simulink model "sixth_harmonic_makale"  (R2013a)
settings: Solver=ode4  StartTime=0.0  StopTime=0.5  FixedStep=Ts  RelTol=1e-3
values from neighbouring files (symbols this model uses):
  Lload = Xload/wout_fund    [acemp_sixth.m]    (also in immd_base_varyingmod.m = Xload/wout; immd_design_elen.m = Xload/wout; immd_efficiency.m = Xload/wout; immd_simulation_base.m = Xload/wout)
  ma1 = 0.8    [acemp_sixth.m]
  ma3 = 0.3    [acemp_sixth.m]
  Rload = Zload*pf    [acemp_sixth.m]    (also in immd_base_varyingmod.m; immd_design_elen.m; immd_efficiency.m; immd_simulation_base.m)
  Ts = 1e-6    (= 1e-06)    [acemp_sixth.m]    (also in immd_base_varyingmod.m = 1e-05; immd_design_elen.m; immd_efficiency.m; immd_simulation_base.m)
  wout_fund = 2*pi*fout_fund    (= 314.159265359)    [acemp_sixth.m]
  wout_three = 2*pi*fout_three    (= 942.477796077)    [acemp_sixth.m]
undefined symbols (not defined in the file or in its folder): phase3, phasegrid
libraries: powerlib x84, powerlib_meascontrol x61, simulink x2
settings Model: Creator=ugurm  LastModifiedBy=ugurm

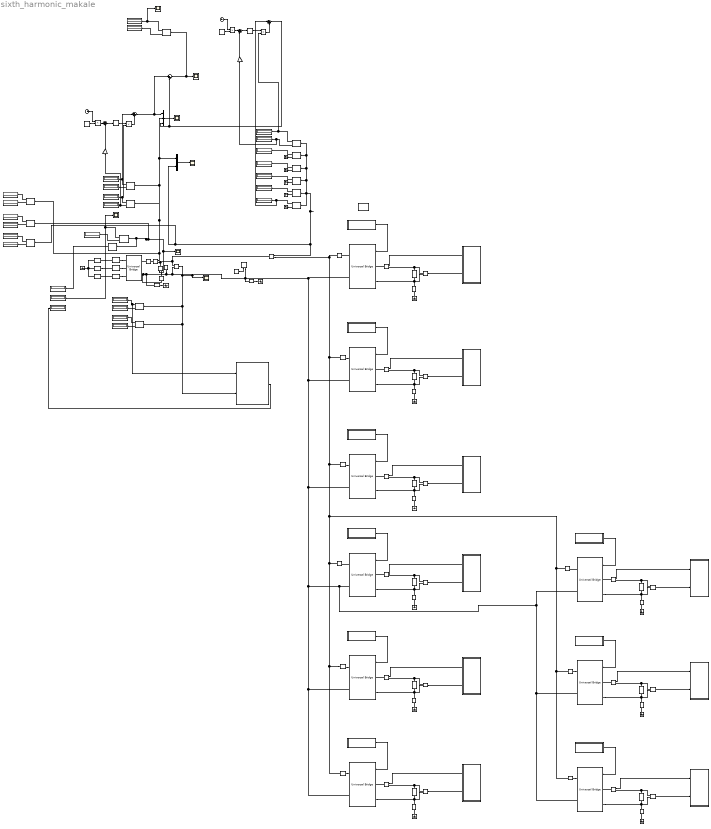
== system sixth_harmonic_makale ==
  AC Voltage Source : powerlib/Electrical Sources/AC Voltage Source  Amplitude=230*sqrt(2)  Phase=phasegrid  Frequency=50  SampleTime=Ts  Measurements=None
  AC Voltage Source1 : powerlib/Electrical Sources/AC Voltage Source  Amplitude=230*sqrt(2)  Phase=-120+phasegrid  Frequency=50  SampleTime=Ts  Measurements=None
  AC Voltage Source2 : powerlib/Electrical Sources/AC Voltage Source  Amplitude=230*sqrt(2)  Phase=120+phasegrid  Frequency=50  SampleTime=Ts  Measurements=None
  Clock : Clock
  Clock1 : Clock
  Constant : Constant  Value=2*pi*300
  Constant1 : Constant  Value=538
  Constant2 : Constant  Value=2*pi*300
  Display{1..20,23,26..28} (24 alike) : Display
  Fourier1 : powerlib_meascontrol/Measurements/Fourier  Freq=50  n=0  InInit=[0, 0]  Ts=Ts
  Fourier10 : powerlib_meascontrol/Measurements/Fourier  Freq=fout_fund  n=6  InInit=[0, 0]  Ts=Ts
  Fourier11 : powerlib_meascontrol/Measurements/Fourier  Freq=50  n=2  InInit=[0, 0]  Ts=Ts
  Fourier12 : powerlib_meascontrol/Measurements/Fourier  Freq=50  n=2  InInit=[0, 0]  Ts=Ts
  Fourier13 : powerlib_meascontrol/Measurements/Fourier  Freq=50  n=0  InInit=[0, 0]  Ts=Ts
  Fourier14 : powerlib_meascontrol/Measurements/Fourier  Freq=50  n=2  InInit=[0, 0]  Ts=Ts
  Fourier15 : powerlib_meascontrol/Measurements/Fourier  Freq=50  n=6  InInit=[0, 0]  Ts=Ts
  Fourier2 : powerlib_meascontrol/Measurements/Fourier  Freq=50  n=6  InInit=[0, 0]  Ts=Ts
  Fourier3 : powerlib_meascontrol/Measurements/Fourier  Freq=fout_fund  n=6  InInit=[0, 0]  Ts=Ts
  Fourier4 : powerlib_meascontrol/Measurements/Fourier  Freq=fout_fund  n=1  InInit=[0, 0]  Ts=Ts
  Fourier5 : powerlib_meascontrol/Measurements/Fourier  Freq=fout_fund  n=0  InInit=[0, 0]  Ts=Ts
  Fourier6 : powerlib_meascontrol/Measurements/Fourier  Freq=fout_fund  n=3  InInit=[0, 0]  Ts=Ts
  Fourier7 : powerlib_meascontrol/Measurements/Fourier  Freq=fout_fund  n=2  InInit=[0, 0]  Ts=Ts
  Fourier8 : powerlib_meascontrol/Measurements/Fourier  Freq=fout_fund  n=6  InInit=[0, 0]  Ts=Ts
  Fourier9 : powerlib_meascontrol/Measurements/Fourier  Freq=fout_fund  n=4  InInit=[0, 0]  Ts=Ts
  Gain : Gain  Gain=pi/180
  Gain1 : Gain  Gain=pi/180
  Gate drive 1 : Subsystem
  Gate drive 2 : Subsystem
  Gate drive 3 : Subsystem
  Gate drive 4 : Subsystem
  Gate drive 5 : Subsystem
  Gate drive 6 : Subsystem
  Gate drive 7 : Subsystem
  Gate drive 8 : Subsystem
  Gate drive 9 : Subsystem
  Ground{1..12} (12 alike) : powerlib/Elements/Ground  LConnTagsString=a
  Idc_m{1..21} (21 alike) : powerlib/Measurements/Current Measurement  PhasorSimulation=off  OutputType=Complex  PSBequivalent=0
  Mux1 : Mux  Inputs=3
  Mux2 : Mux  Inputs=2
  Product{,1..3} (4 alike) : Product
  RMS : powerlib_meascontrol/Measurements/RMS  TrueRMS=on  Freq=50  RMSInit=0  Ts=0
  Scope{1..7} (7 alike) : Scope
      Scope1 settings: YMin=-25  YMax=50  SaveName=idc1
      Scope2 settings: YMin=52.5  YMax=100  SaveName=idc
      Scope3 settings: YMin=0  YMax=100  SaveName=idc2
      Scope4 settings: YMin=440  YMax=650  SaveName=makalee
      Scope5 settings: YMin=0  YMax=25  SaveName=idc4
      Scope6 settings: YMin=0  YMax=25  SaveName=idc5
      Scope7 settings: YMin=440  YMax=650  SaveName=makalee1
  Series RLC Branch{1..2,5,7..8,12..14,17,24..25} (11 alike) : powerlib/Elements/Series RLC Branch  LConnTagsString=__new0  RConnTagsString=__new0  BranchType=R  Resistance=1e12  Inductance=Lload  SetiL0=off  InitialCurrent=0  Capacitance=1e-6  Setx0=off  InitialVoltage=0  Measurements=None
  Series RLC Branch{3..4,6,9..11,22..23,26} (9 alike) : powerlib/Elements/Series RLC Branch  LConnTagsString=__new0  RConnTagsString=__new0  BranchType=RL  Resistance=Rload  Inductance=Lload  SetiL0=off  InitialCurrent=0  Capacitance=1e-6  Setx0=off  InitialVoltage=0  Measurements=None
  Series RLC Branch15 : powerlib/Elements/Series RLC Branch  LConnTagsString=__new0  RConnTagsString=__new0  BranchType=R  Resistance=22.97  Inductance=Lload  SetiL0=off  InitialCurrent=0  Capacitance=1e-6  Setx0=off  InitialVoltage=0  Measurements=None
  Series RLC Branch16 : powerlib/Elements/Series RLC Branch  LConnTagsString=__new0  RConnTagsString=__new0  BranchType=RC  Resistance=1e-9  Inductance=Lload  SetiL0=off  InitialCurrent=0  Capacitance=2e-3  Setx0=off  InitialVoltage=0  Measurements=None
  Series RLC Branch18 : powerlib/Elements/Series RLC Branch  LConnTagsString=__new0  RConnTagsString=__new0  BranchType=RL  Resistance=1e-6  Inductance=1e-9  SetiL0=off  InitialCurrent=0  Capacitance=100e-6  Setx0=off  InitialVoltage=0  Measurements=None
  Series RLC Branch19 : powerlib/Elements/Series RLC Branch  LConnTagsString=__new0  RConnTagsString=__new0  BranchType=RL  Resistance=1e-6  Inductance=1e-9  SetiL0=off  InitialCurrent=0  Capacitance=100e-6  Setx0=off  InitialVoltage=0  Measurements=None
  Series RLC Branch20 : powerlib/Elements/Series RLC Branch  LConnTagsString=__new0  RConnTagsString=__new0  BranchType=RL  Resistance=1e-6  Inductance=1e-9  SetiL0=off  InitialCurrent=0  Capacitance=100e-6  Setx0=off  InitialVoltage=0  Measurements=None
  Series RLC Branch21 : powerlib/Elements/Series RLC Branch  LConnTagsString=__new0  RConnTagsString=__new0  BranchType=RL  Resistance=1e-6  Inductance=1e-3  SetiL0=off  InitialCurrent=0  Capacitance=100e-6  Setx0=off  InitialVoltage=0  Measurements=None
  Subsystem : Subsystem
  Subsystem1 : Subsystem
  Subsystem2 : Subsystem
  Subsystem3 : Subsystem
  Subsystem4 : Subsystem
  Subsystem5 : Subsystem
  Subsystem6 : Subsystem
  Subsystem7 : Subsystem
  Subsystem8 : Subsystem
  Subsystem9 : Subsystem
  Sum{,1..3} (4 alike) : Sum  Inputs=|++
  Sum4 : Sum  Inputs=|+-
  Terminator{4..7,9} (5 alike) : Terminator
  Trigonometric Function : Trigonometry
  Trigonometric Function1 : Trigonometry
  Universal Bridge{1,3..10} (9 alike) : powerlib/Power Electronics/Universal Bridge  Arms=2  SnubberResistance=1e5  SnubberCapacitance=inf  Device=IGBT / Diodes  Ron=1e-6  Lon=0  ForwardVoltages="[  0  0  ]"  ForwardVoltage=0  GTOparameters=[ 10e-6 , 20e-6 ]  IGBTparameters=[0,0]  Measurements=None  Measurements_2=None  converterType=Rectifier
  Universal Bridge2 : powerlib/Power Electronics/Universal Bridge  Arms=3  SnubberResistance=1e5  SnubberCapacitance=inf  Device=Diodes  Ron=1e-6  Lon=0  ForwardVoltages="[  0  0  ]"  ForwardVoltage=0  GTOparameters=[ 10e-6 , 20e-6 ]  IGBTparameters=[0,0]  Measurements=None  Measurements_2=None  converterType=Rectifier
  Vdc2 : powerlib/Electrical Sources/Controlled Voltage Source  Initialize=off  Source_Type=DC  Amplitude=200  Phase=0  Frequency=0  Measurements=None
  Vdc_m{1..10} (10 alike) : powerlib/Measurements/Voltage Measurement  PhasorSimulation=off  OutputType=Complex  PSBequivalent=0
  cap_6 : Display
  cap_rms : Display
  perc_rip : Display
  powergui : powerlib/powergui  Priority=1  SimulationMode=Discrete  SolverType=Tustin  SampleTime=Ts  frequency=60  SPID=off  DisableSnubberDevices=off  DisableRonSwitches=off  DisableVfSwitches=off  SwTol=0  Interpol=off  DisplayEquations=off  frequencyindice=0  Pbase=100e6  ErrMax=1e-4  Iterations=50  UnitsV=kV  UnitsW=MW  FunctionMessages=off  echomessages=off  HookPort=off  EnableUseOfTLC=off  x0status=blocks  RestoreLinks=warning  ResistiveCurrentMeasurement=off  Frange=[0:2:500]  Ylog=off  Xlog=on  ShowGrid=off  save=off  variable=ZData  structure=makalee1  ZoomFFT=off  StartTime=0.2  cycles=15  DisplayStyle=3  fundamental=50  FreqAxis=off  MaxFrequency=1000  frequencyindicesteady=1  RmsSteady=1  display=off  Ts=0  methode=off
  wires:
  Gate drive 1/1(gate1) -> Universal Bridge1/1
  Fourier4/1 -> Display1/1
  Fourier4/2 -> Terminator4/1
  Fourier5/2 -> Terminator5/1
  Fourier6/1 -> Display3/1
  Fourier6/2 -> Terminator6/1
  Fourier7/1 -> Display4/1
  Fourier7/2 -> Terminator7/1
  Idc_m7/1 -> Fourier8/1, Fourier9/1, Fourier6/1, Fourier7/1, Fourier5/1, Fourier4/1, Fourier14/1, Mux2/2
  Fourier9/1 -> Display6/1
  Fourier9/2 -> Terminator9/1
  Idc_m2/1 -> Subsystem/1(In1)
  Vdc_m2/1 -> Subsystem/2(In2)
  Gate drive 2/1(gate1) -> Universal Bridge3/1
  Idc_m3/1 -> Subsystem1/1(In1)
  Vdc_m5/1 -> Subsystem1/2(In2)
  Gate drive 4/1(gate1) -> Universal Bridge4/1
  Idc_m9/1 -> Subsystem2/1(In1)
  Vdc_m6/1 -> Subsystem2/2(In2)
  Constant1/1 -> Vdc2/1
  Vdc_m4/1 -> Scope4/1, Fourier13/1, Subsystem3/2(In2), Fourier15/1
  Fourier13/2 -> Display16/1
  Fourier15/1 -> Display28/1
  Fourier15/2 -> Display27/1
  Fourier1/1 -> Sum/1, Display8/1
  Fourier1/2 -> Display7/1
  Fourier2/1 -> Product/2, Display10/1
  Fourier2/2 -> Gain/1, Display9/1
  Mux2/1 -> Scope1/1
  Trigonometric Function/1 -> Product/1
  Product/1 -> Sum/2
  Clock/1 -> Product1/1
  Constant/1 -> Product1/2
  Product1/1 -> Sum1/1
  Gain/1 -> Sum1/2
  Sum1/1 -> Trigonometric Function/1
  Sum/1 -> Sum4/1, Mux1/1
  Mux1/1 -> Scope2/1
  Fourier5/1 -> Sum2/1, Display2/1
  Fourier8/1 -> Product2/2, Display5/1
  Fourier8/2 -> Gain1/1, Display23/1
  Trigonometric Function1/1 -> Product2/1
  Product2/1 -> Sum2/2
  Clock1/1 -> Product3/1
  Constant2/1 -> Product3/2
  Product3/1 -> Sum3/1
  Gain1/1 -> Sum3/2
  Sum3/1 -> Trigonometric Function1/1
  Sum2/1 -> Sum4/2, Mux1/3
  Sum4/1 -> Fourier3/1, Scope3/1
  Fourier3/1 -> Scope5/1, Display12/1
  Fourier3/2 -> Display11/1
  Idc_m5/1 -> Scope7/1, Fourier12/1, RMS/1, Fourier10/1
  Fourier10/1 -> Scope6/1, cap_6/1
  Fourier10/2 -> Display13/1
  RMS/1 -> cap_rms/1
  Fourier13/1 -> Subsystem3/1(In1), Display26/1
  Subsystem3/1(Out1) -> perc_rip/1
  Gate drive 3/1(gate1) -> Universal Bridge5/1
  Idc_m12/1 -> Subsystem4/1(In1)
  Vdc_m1/1 -> Subsystem4/2(In2)
  Gate drive 5/1(gate1) -> Universal Bridge6/1
  Idc_m13/1 -> Subsystem5/1(In1)
  Vdc_m3/1 -> Subsystem5/2(In2)
  Gate drive 6/1(gate1) -> Universal Bridge7/1
  Idc_m15/1 -> Subsystem6/1(In1)
  Vdc_m7/1 -> Subsystem6/2(In2)
  Gate drive 7/1(gate1) -> Universal Bridge8/1
  Idc_m17/1 -> Subsystem7/1(In1)
  Vdc_m8/1 -> Subsystem7/2(In2)
  Gate drive 8/1(gate1) -> Universal Bridge9/1
  Idc_m18/1 -> Subsystem8/1(In1)
  Vdc_m9/1 -> Subsystem8/2(In2)
  Gate drive 9/1(gate1) -> Universal Bridge10/1
  Idc_m20/1 -> Subsystem9/1(In1)
  Vdc_m10/1 -> Subsystem9/2(In2)
  Idc_m4/1 -> Fourier11/1, Fourier2/1, Mux1/2, Mux2/1, Fourier1/1
  Fourier11/2 -> Display14/1
  Fourier11/1 -> Display15/1
  Fourier12/2 -> Display17/1
  Fourier12/1 -> Display18/1
  Fourier14/2 -> Display19/1
  Fourier14/1 -> Display20/1
  connections:
  Universal Bridge1/RConn1 -- Idc_m1/RConn1
  Universal Bridge1/LConn2 -- Series RLC Branch2/LConn1 -- Vdc_m2/LConn2 -- Series RLC Branch6/RConn1
  Idc_m2/LConn1 -- Universal Bridge1/LConn1
  Series RLC Branch6/LConn1 -- Vdc_m2/LConn1 -- Idc_m2/RConn1
  Ground2/LConn1 -- Series RLC Branch2/RConn1
  Series RLC Branch10/RConn1 -- Series RLC Branch7/LConn1 -- Universal Bridge3/LConn2 -- Vdc_m5/LConn2
  Series RLC Branch10/LConn1 -- Vdc_m5/LConn1 -- Idc_m3/RConn1
  Ground1/LConn1 -- Series RLC Branch7/RConn1
  Idc_m3/LConn1 -- Universal Bridge3/LConn1
  Idc_m6/RConn1 -- Universal Bridge3/RConn1
  Series RLC Branch11/RConn1 -- Series RLC Branch12/LConn1 -- Universal Bridge4/LConn2 -- Vdc_m6/LConn2
  Series RLC Branch11/LConn1 -- Vdc_m6/LConn1 -- Idc_m9/RConn1
  Ground3/LConn1 -- Series RLC Branch12/RConn1
  Idc_m9/LConn1 -- Universal Bridge4/LConn1
  Idc_m11/RConn1 -- Universal Bridge4/RConn1
  Series RLC Branch1/RConn1 -- Ground4/LConn1
  Ground6/LConn1 -- AC Voltage Source2/LConn1 -- AC Voltage Source/LConn1 -- AC Voltage Source1/LConn1
  Series RLC Branch17/RConn1 -- Ground7/LConn1
  Series RLC Branch20/RConn1 -- AC Voltage Source2/RConn1
  AC Voltage Source1/RConn1 -- Series RLC Branch19/RConn1
  Series RLC Branch18/RConn1 -- AC Voltage Source/RConn1
  Series RLC Branch18/LConn1 -- Universal Bridge2/LConn1
  Series RLC Branch19/LConn1 -- Universal Bridge2/LConn2
  Series RLC Branch20/LConn1 -- Universal Bridge2/LConn3
  Vdc_m4/LConn1 -- Idc_m5/LConn1 -- Idc_m4/RConn1 -- Idc_m7/LConn1
  Series RLC Branch21/RConn1 -- Universal Bridge2/RConn1
  Idc_m4/LConn1 -- Series RLC Branch21/LConn1
  Idc_m5/RConn1 -- Series RLC Branch16/LConn1
  Series RLC Branch9/RConn1 -- Universal Bridge5/LConn2 -- Series RLC Branch8/LConn1 -- Vdc_m1/LConn2
  Idc_m12/RConn1 -- Series RLC Branch9/LConn1 -- Vdc_m1/LConn1
  Vdc_m3/LConn2 -- Series RLC Branch3/RConn1 -- Series RLC Branch13/LConn1 -- Universal Bridge6/LConn2
  Idc_m13/RConn1 -- Series RLC Branch3/LConn1 -- Vdc_m3/LConn1
  Vdc_m7/LConn2 -- Series RLC Branch4/RConn1 -- Series RLC Branch5/LConn1 -- Universal Bridge7/LConn2
  Idc_m15/RConn1 -- Series RLC Branch4/LConn1 -- Vdc_m7/LConn1
  Ground9/LConn1 -- Series RLC Branch5/RConn1
  Universal Bridge5/RConn1 -- Idc_m8/RConn1
  Ground5/LConn1 -- Series RLC Branch13/RConn1
  Ground8/LConn1 -- Series RLC Branch8/RConn1
  Idc_m12/LConn1 -- Universal Bridge5/LConn1
  Idc_m15/LConn1 -- Universal Bridge7/LConn1
  Idc_m13/LConn1 -- Universal Bridge6/LConn1
  Idc_m14/RConn1 -- Universal Bridge6/RConn1
  Idc_m10/RConn1 -- Universal Bridge7/RConn1
  Idc_m14/LConn1 -- Idc_m8/LConn1 -- Idc_m16/LConn1 -- Idc_m19/LConn1 -- Idc_m21/LConn1 -- Idc_m1/LConn1 -- Idc_m7/RConn1 -- Idc_m6/LConn1 -- Idc_m11/LConn1 -- Idc_m10/LConn1
  Universal Bridge7/RConn2 -- Universal Bridge8/RConn2 -- Universal Bridge9/RConn2 -- Universal Bridge10/RConn2 -- Universal Bridge5/RConn2 -- Universal Bridge3/RConn2 -- Series RLC Branch15/LConn1 -- Series RLC Branch16/RConn1 -- Universal Bridge2/RConn2 -- Series RLC Branch17/LConn1 -- Vdc_m4/LConn2 -- Series RLC Branch1/LConn1 -- Vdc2/LConn1 -- Universal Bridge1/RConn2 -- Universal Bridge4/RConn2 -- Universal Bridge6/RConn2
  Series RLC Branch26/RConn1 -- Universal Bridge8/LConn2 -- Series RLC Branch25/LConn1 -- Vdc_m8/LConn2
  Idc_m17/RConn1 -- Series RLC Branch26/LConn1 -- Vdc_m8/LConn1
  Vdc_m9/LConn2 -- Series RLC Branch22/RConn1 -- Series RLC Branch14/LConn1 -- Universal Bridge9/LConn2
  Idc_m18/RConn1 -- Series RLC Branch22/LConn1 -- Vdc_m9/LConn1
  Vdc_m10/LConn2 -- Series RLC Branch23/RConn1 -- Series RLC Branch24/LConn1 -- Universal Bridge10/LConn2
  Idc_m20/RConn1 -- Series RLC Branch23/LConn1 -- Vdc_m10/LConn1
  Idc_m17/LConn1 -- Universal Bridge8/LConn1
  Universal Bridge8/RConn1 -- Idc_m21/RConn1
  Idc_m16/RConn1 -- Universal Bridge10/RConn1
  Idc_m19/RConn1 -- Universal Bridge9/RConn1
  Ground10/LConn1 -- Series RLC Branch14/RConn1
  Idc_m18/LConn1 -- Universal Bridge9/LConn1
  Idc_m20/LConn1 -- Universal Bridge10/LConn1
  Ground11/LConn1 -- Series RLC Branch25/RConn1
  Ground12/LConn1 -- Series RLC Branch24/RConn1

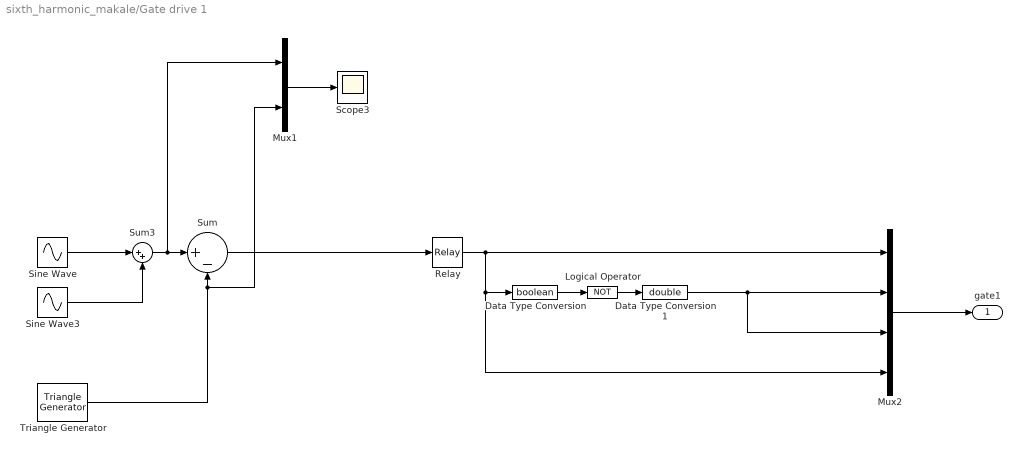
== system sixth_harmonic_makale/Gate drive 1 ==
  Data Type Conversion : DataTypeConversion  OutDataTypeStr=boolean
  Data Type Conversion1 : DataTypeConversion  OutDataTypeStr=double
  Logical Operator : Logic  Operator=NOT  AllPortsSameDT=off  OutDataTypeStr=boolean
  Mux1 : Mux  Inputs=2
  Mux2 : Mux
  Relay : Relay
  Scope3 : Scope
      settings: YMin=-1.75  YMax=1.75  SaveName=idc6
  Sine Wave : Sin  Amplitude=ma1  Frequency=wout_fund  SampleTime=0
  Sine Wave3 : Sin  Amplitude=ma3  Frequency=wout_three  Phase=phase3  SampleTime=0
  Sum : Sum  Inputs=|+-
  Sum3 : Sum  Inputs=|++
  Triangle Generator : powerlib_meascontrol/Pulse & Signal Generators/Triangle Generator  Freq=fsw  Phase=0  Ts=Ts
  gate1 : Outport
  wires:
  Sum/1 -> Relay/1
  Data Type Conversion/1 -> Logical Operator/1
  Relay/1 -> Mux2/4, Data Type Conversion/1, Mux2/1
  Logical Operator/1 -> Data Type Conversion1/1
  Data Type Conversion1/1 -> Mux2/2, Mux2/3
  Mux2/1 -> gate1/1
  Sine Wave/1 -> Sum3/1
  Sine Wave3/1 -> Sum3/2
  Sum3/1 -> Mux1/1, Sum/1
  Triangle Generator/1 -> Mux1/2, Sum/2
  Mux1/1 -> Scope3/1

== system sixth_harmonic_makale/Gate drive 2 ==
  Data Type Conversion : DataTypeConversion  OutDataTypeStr=boolean
  Data Type Conversion1 : DataTypeConversion  OutDataTypeStr=double
  Logical Operator : Logic  Operator=NOT  AllPortsSameDT=off  OutDataTypeStr=boolean
  Mux1 : Mux  Inputs=2
  Mux2 : Mux
  Relay : Relay
  Scope3 : Scope
      settings: YMin=-1.75  YMax=1.75  SaveName=idc7
  Sine Wave : Sin  Amplitude=ma1  Frequency=wout_fund  Phase=-2*pi/3  SampleTime=0
  Sine Wave3 : Sin  Amplitude=ma3  Frequency=wout_three  Phase=phase3  SampleTime=0
  Sum : Sum  Inputs=|+-
  Sum3 : Sum  Inputs=|++
  Triangle Generator : powerlib_meascontrol/Pulse & Signal Generators/Triangle Generator  Freq=fsw  Phase=0  Ts=Ts
  gate1 : Outport
  wires:
  Sum/1 -> Relay/1
  Data Type Conversion/1 -> Logical Operator/1
  Relay/1 -> Mux2/4, Data Type Conversion/1, Mux2/1
  Logical Operator/1 -> Data Type Conversion1/1
  Data Type Conversion1/1 -> Mux2/2, Mux2/3
  Mux2/1 -> gate1/1
  Sum3/1 -> Mux1/1, Sum/1
  Triangle Generator/1 -> Mux1/2, Sum/2
  Sine Wave/1 -> Sum3/1
  Sine Wave3/1 -> Sum3/2
  Mux1/1 -> Scope3/1

== system sixth_harmonic_makale/Gate drive 3 ==
  Data Type Conversion : DataTypeConversion  OutDataTypeStr=boolean
  Data Type Conversion1 : DataTypeConversion  OutDataTypeStr=double
  Logical Operator : Logic  Operator=NOT  AllPortsSameDT=off  OutDataTypeStr=boolean
  Mux1 : Mux  Inputs=2
  Mux2 : Mux
  Relay : Relay
  Scope3 : Scope
      settings: YMin=-1.75  YMax=1.75  SaveName=idc6
  Sine Wave : Sin  Amplitude=ma1  Frequency=wout_fund  SampleTime=0
  Sine Wave3 : Sin  Amplitude=ma3  Frequency=wout_three  Phase=phase3  SampleTime=0
  Sum : Sum  Inputs=|+-
  Sum3 : Sum  Inputs=|++
  Triangle Generator : powerlib_meascontrol/Pulse & Signal Generators/Triangle Generator  Freq=fsw  Phase=0  Ts=Ts
  gate1 : Outport
  wires:
  Sum/1 -> Relay/1
  Data Type Conversion/1 -> Logical Operator/1
  Relay/1 -> Mux2/4, Data Type Conversion/1, Mux2/1
  Logical Operator/1 -> Data Type Conversion1/1
  Data Type Conversion1/1 -> Mux2/2, Mux2/3
  Mux2/1 -> gate1/1
  Sine Wave/1 -> Sum3/1
  Sine Wave3/1 -> Sum3/2
  Sum3/1 -> Mux1/1, Sum/1
  Triangle Generator/1 -> Mux1/2, Sum/2
  Mux1/1 -> Scope3/1

== system sixth_harmonic_makale/Gate drive 4 ==
  Data Type Conversion : DataTypeConversion  OutDataTypeStr=boolean
  Data Type Conversion1 : DataTypeConversion  OutDataTypeStr=double
  Logical Operator : Logic  Operator=NOT  AllPortsSameDT=off  OutDataTypeStr=boolean
  Mux1 : Mux  Inputs=2
  Mux2 : Mux
  Relay : Relay
  Scope3 : Scope
      settings: YMin=-1.75  YMax=1.75  SaveName=idc8
  Sine Wave : Sin  Amplitude=ma1  Frequency=wout_fund  Phase=-4*pi/3  SampleTime=0
  Sine Wave3 : Sin  Amplitude=ma3  Frequency=wout_three  Phase=phase3  SampleTime=0
  Sum : Sum  Inputs=|+-
  Sum3 : Sum  Inputs=|++
  Triangle Generator : powerlib_meascontrol/Pulse & Signal Generators/Triangle Generator  Freq=fsw  Phase=0  Ts=Ts
  gate1 : Outport
  wires:
  Sum/1 -> Relay/1
  Data Type Conversion/1 -> Logical Operator/1
  Relay/1 -> Mux2/4, Data Type Conversion/1, Mux2/1
  Logical Operator/1 -> Data Type Conversion1/1
  Data Type Conversion1/1 -> Mux2/2, Mux2/3
  Mux2/1 -> gate1/1
  Sum3/1 -> Mux1/1, Sum/1
  Triangle Generator/1 -> Mux1/2, Sum/2
  Sine Wave/1 -> Sum3/1
  Sine Wave3/1 -> Sum3/2
  Mux1/1 -> Scope3/1

== system sixth_harmonic_makale/Gate drive 5 ==
  Data Type Conversion : DataTypeConversion  OutDataTypeStr=boolean
  Data Type Conversion1 : DataTypeConversion  OutDataTypeStr=double
  Logical Operator : Logic  Operator=NOT  AllPortsSameDT=off  OutDataTypeStr=boolean
  Mux2 : Mux
  Relay : Relay
  Sine Wave : Sin  Amplitude=ma1  Frequency=wout_fund  Phase=-2*pi/3  SampleTime=0
  Sine Wave3 : Sin  Amplitude=ma3  Frequency=wout_three  Phase=phase3  SampleTime=0
  Sum : Sum  Inputs=|+-
  Sum3 : Sum  Inputs=|++
  Triangle Generator : powerlib_meascontrol/Pulse & Signal Generators/Triangle Generator  Freq=fsw  Phase=0  Ts=Ts
  gate1 : Outport
  wires:
  Sum/1 -> Relay/1
  Data Type Conversion/1 -> Logical Operator/1
  Relay/1 -> Mux2/4, Data Type Conversion/1, Mux2/1
  Logical Operator/1 -> Data Type Conversion1/1
  Data Type Conversion1/1 -> Mux2/2, Mux2/3
  Mux2/1 -> gate1/1
  Sine Wave/1 -> Sum3/1
  Sine Wave3/1 -> Sum3/2
  Sum3/1 -> Sum/1
  Triangle Generator/1 -> Sum/2

== system sixth_harmonic_makale/Gate drive 6 ==
  Data Type Conversion : DataTypeConversion  OutDataTypeStr=boolean
  Data Type Conversion1 : DataTypeConversion  OutDataTypeStr=double
  Logical Operator : Logic  Operator=NOT  AllPortsSameDT=off  OutDataTypeStr=boolean
  Mux2 : Mux
  Relay : Relay
  Sine Wave : Sin  Amplitude=ma1  Frequency=wout_fund  Phase=-4*pi/3  SampleTime=0
  Sine Wave3 : Sin  Amplitude=ma3  Frequency=wout_three  Phase=phase3  SampleTime=0
  Sum : Sum  Inputs=|+-
  Sum3 : Sum  Inputs=|++
  Triangle Generator : powerlib_meascontrol/Pulse & Signal Generators/Triangle Generator  Freq=fsw  Phase=0  Ts=Ts
  gate1 : Outport
  wires:
  Sum/1 -> Relay/1
  Data Type Conversion/1 -> Logical Operator/1
  Relay/1 -> Mux2/4, Data Type Conversion/1, Mux2/1
  Logical Operator/1 -> Data Type Conversion1/1
  Data Type Conversion1/1 -> Mux2/2, Mux2/3
  Mux2/1 -> gate1/1
  Sine Wave/1 -> Sum3/1
  Sine Wave3/1 -> Sum3/2
  Sum3/1 -> Sum/1
  Triangle Generator/1 -> Sum/2

== system sixth_harmonic_makale/Gate drive 7 ==
  Data Type Conversion : DataTypeConversion  OutDataTypeStr=boolean
  Data Type Conversion1 : DataTypeConversion  OutDataTypeStr=double
  Logical Operator : Logic  Operator=NOT  AllPortsSameDT=off  OutDataTypeStr=boolean
  Mux1 : Mux  Inputs=2
  Mux2 : Mux
  Relay : Relay
  Scope3 : Scope
      settings: YMin=-1.75  YMax=1.75  SaveName=idc6
  Sine Wave : Sin  Amplitude=ma1  Frequency=wout_fund  SampleTime=0
  Sine Wave3 : Sin  Amplitude=ma3  Frequency=wout_three  Phase=phase3  SampleTime=0
  Sum : Sum  Inputs=|+-
  Sum3 : Sum  Inputs=|++
  Triangle Generator : powerlib_meascontrol/Pulse & Signal Generators/Triangle Generator  Freq=fsw  Phase=0  Ts=Ts
  gate1 : Outport
  wires:
  Sum/1 -> Relay/1
  Data Type Conversion/1 -> Logical Operator/1
  Relay/1 -> Mux2/4, Data Type Conversion/1, Mux2/1
  Logical Operator/1 -> Data Type Conversion1/1
  Data Type Conversion1/1 -> Mux2/2, Mux2/3
  Mux2/1 -> gate1/1
  Sine Wave/1 -> Sum3/1
  Sine Wave3/1 -> Sum3/2
  Sum3/1 -> Mux1/1, Sum/1
  Triangle Generator/1 -> Mux1/2, Sum/2
  Mux1/1 -> Scope3/1

== system sixth_harmonic_makale/Gate drive 8 ==
  Data Type Conversion : DataTypeConversion  OutDataTypeStr=boolean
  Data Type Conversion1 : DataTypeConversion  OutDataTypeStr=double
  Logical Operator : Logic  Operator=NOT  AllPortsSameDT=off  OutDataTypeStr=boolean
  Mux2 : Mux
  Relay : Relay
  Sine Wave : Sin  Amplitude=ma1  Frequency=wout_fund  Phase=-2*pi/3  SampleTime=0
  Sine Wave3 : Sin  Amplitude=ma3  Frequency=wout_three  Phase=phase3  SampleTime=0
  Sum : Sum  Inputs=|+-
  Sum3 : Sum  Inputs=|++
  Triangle Generator : powerlib_meascontrol/Pulse & Signal Generators/Triangle Generator  Freq=fsw  Phase=0  Ts=Ts
  gate1 : Outport
  wires:
  Sum/1 -> Relay/1
  Data Type Conversion/1 -> Logical Operator/1
  Relay/1 -> Mux2/4, Data Type Conversion/1, Mux2/1
  Logical Operator/1 -> Data Type Conversion1/1
  Data Type Conversion1/1 -> Mux2/2, Mux2/3
  Mux2/1 -> gate1/1
  Sine Wave/1 -> Sum3/1
  Sine Wave3/1 -> Sum3/2
  Sum3/1 -> Sum/1
  Triangle Generator/1 -> Sum/2

== system sixth_harmonic_makale/Gate drive 9 ==
  Data Type Conversion : DataTypeConversion  OutDataTypeStr=boolean
  Data Type Conversion1 : DataTypeConversion  OutDataTypeStr=double
  Logical Operator : Logic  Operator=NOT  AllPortsSameDT=off  OutDataTypeStr=boolean
  Mux2 : Mux
  Relay : Relay
  Sine Wave : Sin  Amplitude=ma1  Frequency=wout_fund  Phase=-4*pi/3  SampleTime=0
  Sine Wave3 : Sin  Amplitude=ma3  Frequency=wout_three  Phase=phase3  SampleTime=0
  Sum : Sum  Inputs=|+-
  Sum3 : Sum  Inputs=|++
  Triangle Generator : powerlib_meascontrol/Pulse & Signal Generators/Triangle Generator  Freq=fsw  Phase=0  Ts=Ts
  gate1 : Outport
  wires:
  Sum/1 -> Relay/1
  Data Type Conversion/1 -> Logical Operator/1
  Relay/1 -> Mux2/4, Data Type Conversion/1, Mux2/1
  Logical Operator/1 -> Data Type Conversion1/1
  Data Type Conversion1/1 -> Mux2/2, Mux2/3
  Mux2/1 -> gate1/1
  Sine Wave/1 -> Sum3/1
  Sine Wave3/1 -> Sum3/2
  Sum3/1 -> Sum/1
  Triangle Generator/1 -> Sum/2

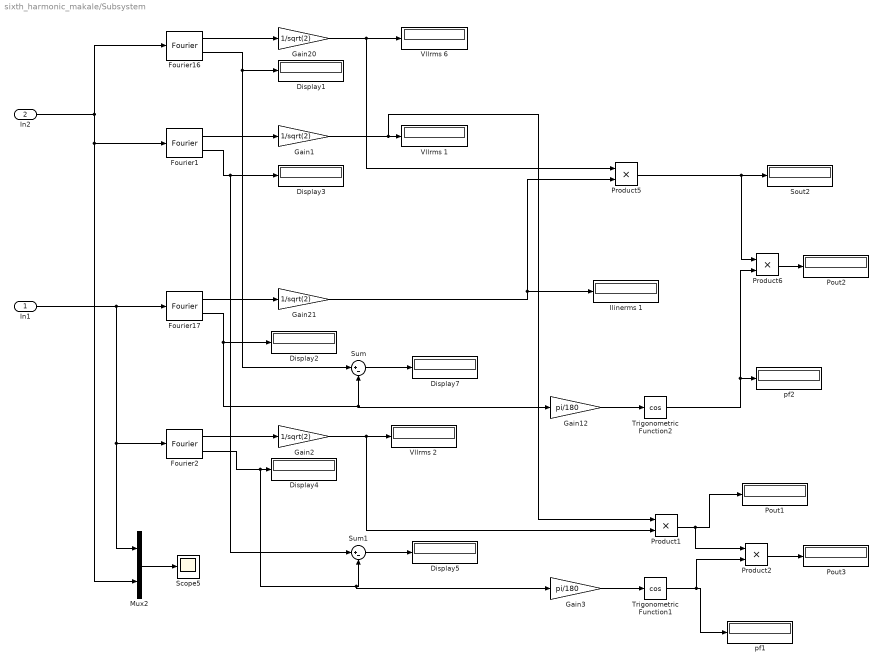
== system sixth_harmonic_makale/Subsystem ==
  In1 : Inport
  In2 : Inport  Port=2
  Display{1..5,7} (6 alike) : Display
  Fourier1 : powerlib_meascontrol/Measurements/Fourier  Freq=fout_fund  n=3  InInit=[0, 0]  Ts=Ts
  Fourier16 : powerlib_meascontrol/Measurements/Fourier  Freq=fout_fund  n=1  InInit=[0, 0]  Ts=Ts
  Fourier17 : powerlib_meascontrol/Measurements/Fourier  Freq=fout_fund  n=1  InInit=[0, 0]  Ts=Ts
  Fourier2 : powerlib_meascontrol/Measurements/Fourier  Freq=fout_fund  n=3  InInit=[0, 0]  Ts=Ts
  Gain{1..2,20..21} (4 alike) : Gain  Gain=1/sqrt(2)
  Gain12 : Gain  Gain=pi/180
  Gain3 : Gain  Gain=pi/180
  Ilinerms 1 : Display
  Mux2 : Mux  Inputs=2
  Pout1 : Display
  Pout2 : Display
  Pout3 : Display
  Product{1..2,5..6} (4 alike) : Product
  Scope5 : Scope
      settings: YMin=-700  YMax=700  SaveName=ScopeData2
  Sout2 : Display
      settings: Format=short_e
  Sum : Sum  Inputs=|+-
  Sum1 : Sum  Inputs=|+-
  Trigonometric Function1 : Trigonometry  Operator=cos
  Trigonometric Function2 : Trigonometry  Operator=cos
  Vllrms 1 : Display
  Vllrms 2 : Display
  Vllrms 6 : Display
  pf1 : Display
  pf2 : Display
  wires:
  Mux2/1 -> Scope5/1
  In2/1 -> Fourier16/1, Fourier1/1, Mux2/2
  In1/1 -> Fourier17/1, Fourier2/1, Mux2/1
  Gain20/1 -> Vllrms 6/1, Product5/1
  Gain21/1 -> Ilinerms 1/1, Product5/2
  Fourier17/1 -> Gain21/1
  Trigonometric Function2/1 -> Product6/2, pf2/1
  Gain12/1 -> Trigonometric Function2/1
  Product6/1 -> Pout2/1
  Fourier16/1 -> Gain20/1
  Product5/1 -> Product6/1, Sout2/1
  Fourier16/2 -> Display1/1, Sum/1
  Fourier17/2 -> Display2/1, Sum/2, Gain12/1
  Sum/1 -> Display7/1
  Fourier1/1 -> Gain1/1
  Gain1/1 -> Product1/1, Vllrms 1/1
  Fourier1/2 -> Display3/1, Sum1/1
  Fourier2/1 -> Gain2/1
  Gain2/1 -> Product1/2, Vllrms 2/1
  Fourier2/2 -> Gain3/1, Sum1/2, Display4/1
  Sum1/1 -> Display5/1
  Gain3/1 -> Trigonometric Function1/1
  Trigonometric Function1/1 -> Product2/2, pf1/1
  Product1/1 -> Product2/1, Pout1/1
  Product2/1 -> Pout3/1

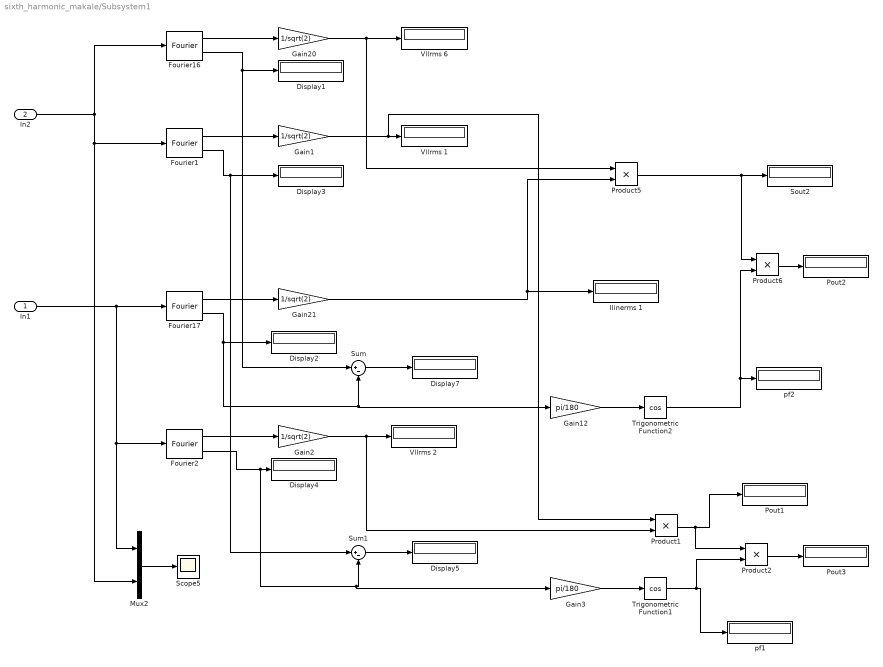
== system sixth_harmonic_makale/Subsystem1 ==
  In1 : Inport
  In2 : Inport  Port=2
  Display{1..5,7} (6 alike) : Display
  Fourier1 : powerlib_meascontrol/Measurements/Fourier  Freq=fout_fund  n=3  InInit=[0, 0]  Ts=Ts
  Fourier16 : powerlib_meascontrol/Measurements/Fourier  Freq=fout_fund  n=1  InInit=[0, 0]  Ts=Ts
  Fourier17 : powerlib_meascontrol/Measurements/Fourier  Freq=fout_fund  n=1  InInit=[0, 0]  Ts=Ts
  Fourier2 : powerlib_meascontrol/Measurements/Fourier  Freq=fout_fund  n=3  InInit=[0, 0]  Ts=Ts
  Gain{1..2,20..21} (4 alike) : Gain  Gain=1/sqrt(2)
  Gain12 : Gain  Gain=pi/180
  Gain3 : Gain  Gain=pi/180
  Ilinerms 1 : Display
  Mux2 : Mux  Inputs=2
  Pout1 : Display
  Pout2 : Display
  Pout3 : Display
  Product{1..2,5..6} (4 alike) : Product
  Scope5 : Scope
      settings: YMin=-700  YMax=700  SaveName=ScopeData2
  Sout2 : Display
      settings: Format=short_e
  Sum : Sum  Inputs=|+-
  Sum1 : Sum  Inputs=|+-
  Trigonometric Function1 : Trigonometry  Operator=cos
  Trigonometric Function2 : Trigonometry  Operator=cos
  Vllrms 1 : Display
  Vllrms 2 : Display
  Vllrms 6 : Display
  pf1 : Display
  pf2 : Display
  wires:
  Mux2/1 -> Scope5/1
  In2/1 -> Fourier16/1, Fourier1/1, Mux2/2
  In1/1 -> Fourier17/1, Fourier2/1, Mux2/1
  Gain20/1 -> Vllrms 6/1, Product5/1
  Gain21/1 -> Ilinerms 1/1, Product5/2
  Fourier17/1 -> Gain21/1
  Trigonometric Function2/1 -> Product6/2, pf2/1
  Gain12/1 -> Trigonometric Function2/1
  Product6/1 -> Pout2/1
  Fourier16/1 -> Gain20/1
  Product5/1 -> Product6/1, Sout2/1
  Fourier16/2 -> Display1/1, Sum/1
  Fourier17/2 -> Display2/1, Sum/2, Gain12/1
  Sum/1 -> Display7/1
  Fourier1/1 -> Gain1/1
  Gain1/1 -> Product1/1, Vllrms 1/1
  Fourier1/2 -> Display3/1, Sum1/1
  Fourier2/1 -> Gain2/1
  Gain2/1 -> Product1/2, Vllrms 2/1
  Fourier2/2 -> Gain3/1, Sum1/2, Display4/1
  Sum1/1 -> Display5/1
  Gain3/1 -> Trigonometric Function1/1
  Trigonometric Function1/1 -> Product2/2, pf1/1
  Product1/1 -> Product2/1, Pout1/1
  Product2/1 -> Pout3/1

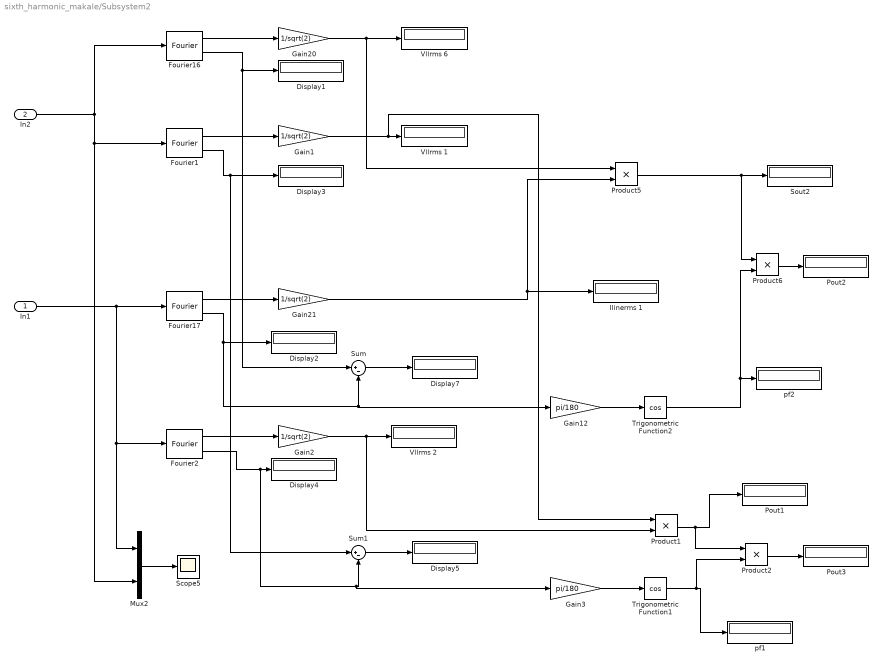
== system sixth_harmonic_makale/Subsystem2 ==
  In1 : Inport
  In2 : Inport  Port=2
  Display{1..5,7} (6 alike) : Display
  Fourier1 : powerlib_meascontrol/Measurements/Fourier  Freq=fout_fund  n=3  InInit=[0, 0]  Ts=Ts
  Fourier16 : powerlib_meascontrol/Measurements/Fourier  Freq=fout_fund  n=1  InInit=[0, 0]  Ts=Ts
  Fourier17 : powerlib_meascontrol/Measurements/Fourier  Freq=fout_fund  n=1  InInit=[0, 0]  Ts=Ts
  Fourier2 : powerlib_meascontrol/Measurements/Fourier  Freq=fout_fund  n=3  InInit=[0, 0]  Ts=Ts
  Gain{1..2,20..21} (4 alike) : Gain  Gain=1/sqrt(2)
  Gain12 : Gain  Gain=pi/180
  Gain3 : Gain  Gain=pi/180
  Ilinerms 1 : Display
  Mux2 : Mux  Inputs=2
  Pout1 : Display
  Pout2 : Display
  Pout3 : Display
  Product{1..2,5..6} (4 alike) : Product
  Scope5 : Scope
      settings: YMin=-700  YMax=700  SaveName=ScopeData2
  Sout2 : Display
      settings: Format=short_e
  Sum : Sum  Inputs=|+-
  Sum1 : Sum  Inputs=|+-
  Trigonometric Function1 : Trigonometry  Operator=cos
  Trigonometric Function2 : Trigonometry  Operator=cos
  Vllrms 1 : Display
  Vllrms 2 : Display
  Vllrms 6 : Display
  pf1 : Display
  pf2 : Display
  wires:
  Mux2/1 -> Scope5/1
  In2/1 -> Fourier16/1, Fourier1/1, Mux2/2
  In1/1 -> Fourier17/1, Fourier2/1, Mux2/1
  Gain20/1 -> Vllrms 6/1, Product5/1
  Gain21/1 -> Ilinerms 1/1, Product5/2
  Fourier17/1 -> Gain21/1
  Trigonometric Function2/1 -> Product6/2, pf2/1
  Gain12/1 -> Trigonometric Function2/1
  Product6/1 -> Pout2/1
  Fourier16/1 -> Gain20/1
  Product5/1 -> Product6/1, Sout2/1
  Fourier16/2 -> Display1/1, Sum/1
  Fourier17/2 -> Display2/1, Sum/2, Gain12/1
  Sum/1 -> Display7/1
  Fourier1/1 -> Gain1/1
  Gain1/1 -> Product1/1, Vllrms 1/1
  Fourier1/2 -> Display3/1, Sum1/1
  Fourier2/1 -> Gain2/1
  Gain2/1 -> Product1/2, Vllrms 2/1
  Fourier2/2 -> Gain3/1, Sum1/2, Display4/1
  Sum1/1 -> Display5/1
  Gain3/1 -> Trigonometric Function1/1
  Trigonometric Function1/1 -> Product2/2, pf1/1
  Product1/1 -> Product2/1, Pout1/1
  Product2/1 -> Pout3/1

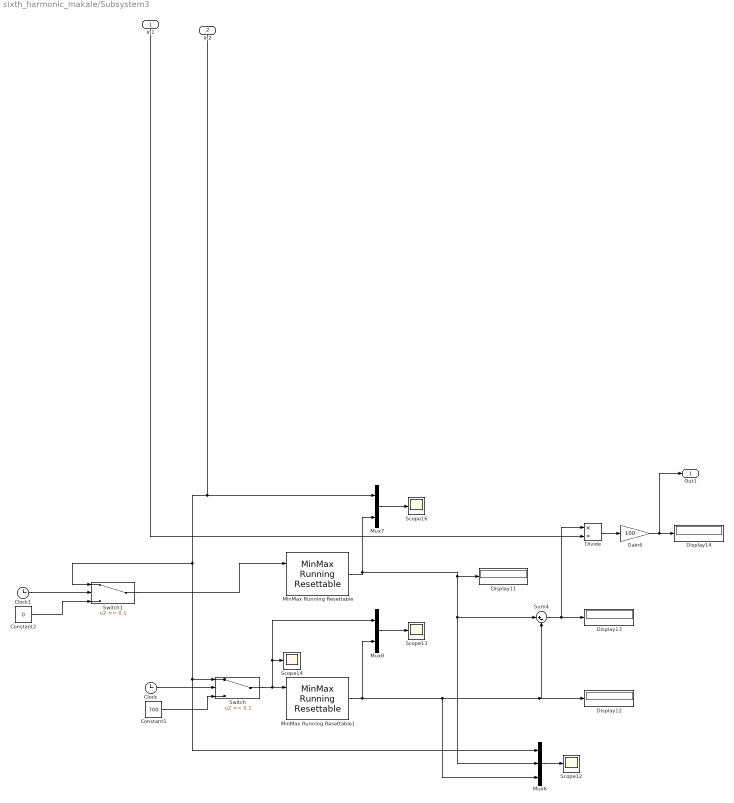
== system sixth_harmonic_makale/Subsystem3 ==
  In1 : Inport
  In2 : Inport  Port=2
  Clock : Clock
  Clock1 : Clock
  Constant1 : Constant  Value=700  SampleTime=Ts
  Constant2 : Constant  Value=0  SampleTime=Ts
  Display{11..14} (4 alike) : Display
  Divide : Product  Inputs=*/
  Gain6 : Gain  Gain=100
  MinMax Running Resettable : simulink/Math Operations/MinMax Running Resettable  Function=max  vinit=0.0
  MinMax Running Resettable1 : simulink/Math Operations/MinMax Running Resettable  Function=min  vinit=700
  Mux6 : Mux  Inputs=3
  Mux7 : Mux  Inputs=2
  Mux8 : Mux  Inputs=2
  Scope{12..14,16} (4 alike) : Scope
      Scope12 settings: YMin=529  YMax=548  SaveName=ScopeData11
      Scope13 settings: YMin=520  YMax=700  SaveName=ScopeData12
      Scope14 settings: YMin=475  YMax=525  SaveName=ScopeData13
      Scope16 settings: YMin=0  YMax=1000  SaveName=ScopeData15
  Sum4 : Sum  Inputs=|+-
  Switch : Switch  Threshold=0.1
  Switch1 : Switch  Threshold=0.1
  Out1 : Outport
  wires:
  MinMax Running Resettable/1 -> Display11/1, Mux6/2, Sum4/1, Mux7/2
  Clock/1 -> Switch/2
  Mux8/1 -> Scope13/1
  Gain6/1 -> Out1/1, Display14/1
  Constant1/1 -> Switch/3
  MinMax Running Resettable1/1 -> Mux6/3, Display12/1, Sum4/2, Mux8/2
  Mux7/1 -> Scope16/1
  Switch/1 -> Mux8/1, Scope14/1, MinMax Running Resettable1/1
  Sum4/1 -> Divide/1, Display13/1
  Divide/1 -> Gain6/1
  Mux6/1 -> Scope12/1
  In1/1 -> Divide/2
  In2/1 -> Mux6/1, Switch/1, Switch1/1, Mux7/1
  Clock1/1 -> Switch1/2
  Constant2/1 -> Switch1/3
  Switch1/1 -> MinMax Running Resettable/1

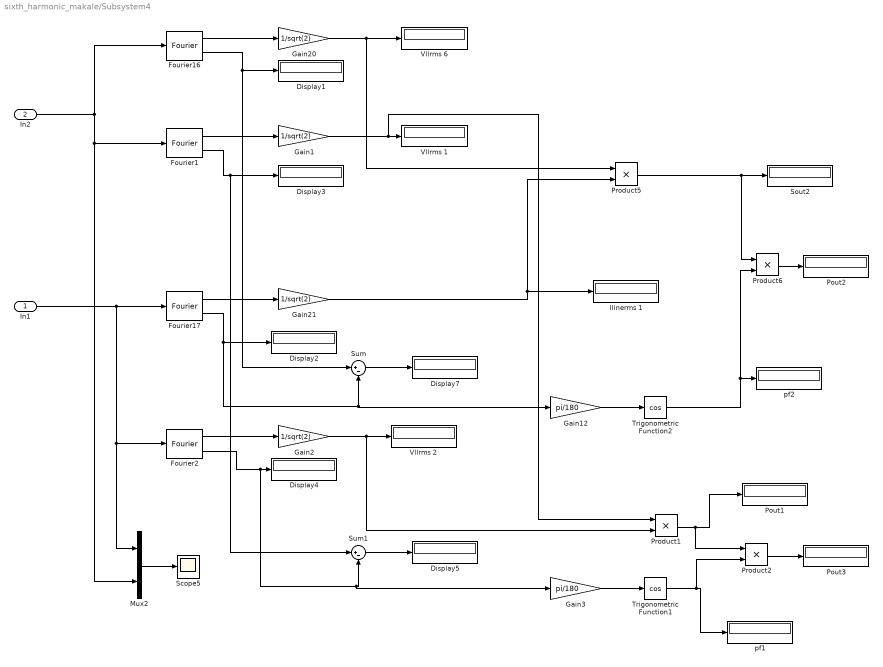
== system sixth_harmonic_makale/Subsystem4 ==
  In1 : Inport
  In2 : Inport  Port=2
  Display{1..5,7} (6 alike) : Display
  Fourier1 : powerlib_meascontrol/Measurements/Fourier  Freq=fout_fund  n=3  InInit=[0, 0]  Ts=Ts
  Fourier16 : powerlib_meascontrol/Measurements/Fourier  Freq=fout_fund  n=1  InInit=[0, 0]  Ts=Ts
  Fourier17 : powerlib_meascontrol/Measurements/Fourier  Freq=fout_fund  n=1  InInit=[0, 0]  Ts=Ts
  Fourier2 : powerlib_meascontrol/Measurements/Fourier  Freq=fout_fund  n=3  InInit=[0, 0]  Ts=Ts
  Gain{1..2,20..21} (4 alike) : Gain  Gain=1/sqrt(2)
  Gain12 : Gain  Gain=pi/180
  Gain3 : Gain  Gain=pi/180
  Ilinerms 1 : Display
  Mux2 : Mux  Inputs=2
  Pout1 : Display
  Pout2 : Display
  Pout3 : Display
  Product{1..2,5..6} (4 alike) : Product
  Scope5 : Scope
      settings: YMin=-700  YMax=700  SaveName=ScopeData2
  Sout2 : Display
      settings: Format=short_e
  Sum : Sum  Inputs=|+-
  Sum1 : Sum  Inputs=|+-
  Trigonometric Function1 : Trigonometry  Operator=cos
  Trigonometric Function2 : Trigonometry  Operator=cos
  Vllrms 1 : Display
  Vllrms 2 : Display
  Vllrms 6 : Display
  pf1 : Display
  pf2 : Display
  wires:
  Mux2/1 -> Scope5/1
  In2/1 -> Fourier16/1, Fourier1/1, Mux2/2
  In1/1 -> Fourier17/1, Fourier2/1, Mux2/1
  Gain20/1 -> Vllrms 6/1, Product5/1
  Gain21/1 -> Ilinerms 1/1, Product5/2
  Fourier17/1 -> Gain21/1
  Trigonometric Function2/1 -> Product6/2, pf2/1
  Gain12/1 -> Trigonometric Function2/1
  Product6/1 -> Pout2/1
  Fourier16/1 -> Gain20/1
  Product5/1 -> Product6/1, Sout2/1
  Fourier16/2 -> Display1/1, Sum/1
  Fourier17/2 -> Display2/1, Sum/2, Gain12/1
  Sum/1 -> Display7/1
  Fourier1/1 -> Gain1/1
  Gain1/1 -> Product1/1, Vllrms 1/1
  Fourier1/2 -> Display3/1, Sum1/1
  Fourier2/1 -> Gain2/1
  Gain2/1 -> Product1/2, Vllrms 2/1
  Fourier2/2 -> Gain3/1, Sum1/2, Display4/1
  Sum1/1 -> Display5/1
  Gain3/1 -> Trigonometric Function1/1
  Trigonometric Function1/1 -> Product2/2, pf1/1
  Product1/1 -> Product2/1, Pout1/1
  Product2/1 -> Pout3/1

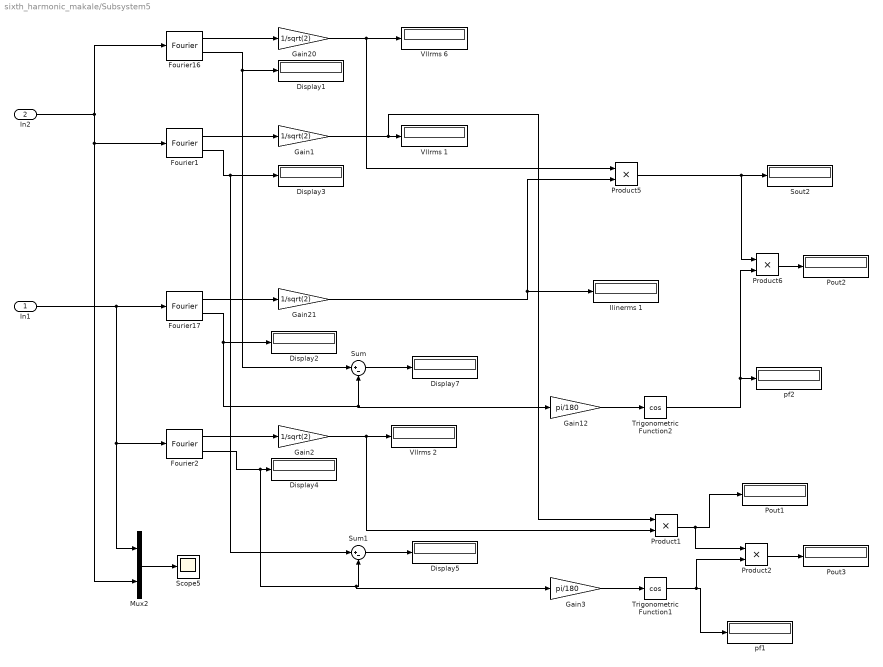
== system sixth_harmonic_makale/Subsystem5 ==
  In1 : Inport
  In2 : Inport  Port=2
  Display{1..5,7} (6 alike) : Display
  Fourier1 : powerlib_meascontrol/Measurements/Fourier  Freq=fout_fund  n=3  InInit=[0, 0]  Ts=Ts
  Fourier16 : powerlib_meascontrol/Measurements/Fourier  Freq=fout_fund  n=1  InInit=[0, 0]  Ts=Ts
  Fourier17 : powerlib_meascontrol/Measurements/Fourier  Freq=fout_fund  n=1  InInit=[0, 0]  Ts=Ts
  Fourier2 : powerlib_meascontrol/Measurements/Fourier  Freq=fout_fund  n=3  InInit=[0, 0]  Ts=Ts
  Gain{1..2,20..21} (4 alike) : Gain  Gain=1/sqrt(2)
  Gain12 : Gain  Gain=pi/180
  Gain3 : Gain  Gain=pi/180
  Ilinerms 1 : Display
  Mux2 : Mux  Inputs=2
  Pout1 : Display
  Pout2 : Display
  Pout3 : Display
  Product{1..2,5..6} (4 alike) : Product
  Scope5 : Scope
      settings: YMin=-700  YMax=700  SaveName=ScopeData2
  Sout2 : Display
      settings: Format=short_e
  Sum : Sum  Inputs=|+-
  Sum1 : Sum  Inputs=|+-
  Trigonometric Function1 : Trigonometry  Operator=cos
  Trigonometric Function2 : Trigonometry  Operator=cos
  Vllrms 1 : Display
  Vllrms 2 : Display
  Vllrms 6 : Display
  pf1 : Display
  pf2 : Display
  wires:
  Mux2/1 -> Scope5/1
  In2/1 -> Fourier16/1, Fourier1/1, Mux2/2
  In1/1 -> Fourier17/1, Fourier2/1, Mux2/1
  Gain20/1 -> Vllrms 6/1, Product5/1
  Gain21/1 -> Ilinerms 1/1, Product5/2
  Fourier17/1 -> Gain21/1
  Trigonometric Function2/1 -> Product6/2, pf2/1
  Gain12/1 -> Trigonometric Function2/1
  Product6/1 -> Pout2/1
  Fourier16/1 -> Gain20/1
  Product5/1 -> Product6/1, Sout2/1
  Fourier16/2 -> Display1/1, Sum/1
  Fourier17/2 -> Display2/1, Sum/2, Gain12/1
  Sum/1 -> Display7/1
  Fourier1/1 -> Gain1/1
  Gain1/1 -> Product1/1, Vllrms 1/1
  Fourier1/2 -> Display3/1, Sum1/1
  Fourier2/1 -> Gain2/1
  Gain2/1 -> Product1/2, Vllrms 2/1
  Fourier2/2 -> Gain3/1, Sum1/2, Display4/1
  Sum1/1 -> Display5/1
  Gain3/1 -> Trigonometric Function1/1
  Trigonometric Function1/1 -> Product2/2, pf1/1
  Product1/1 -> Product2/1, Pout1/1
  Product2/1 -> Pout3/1

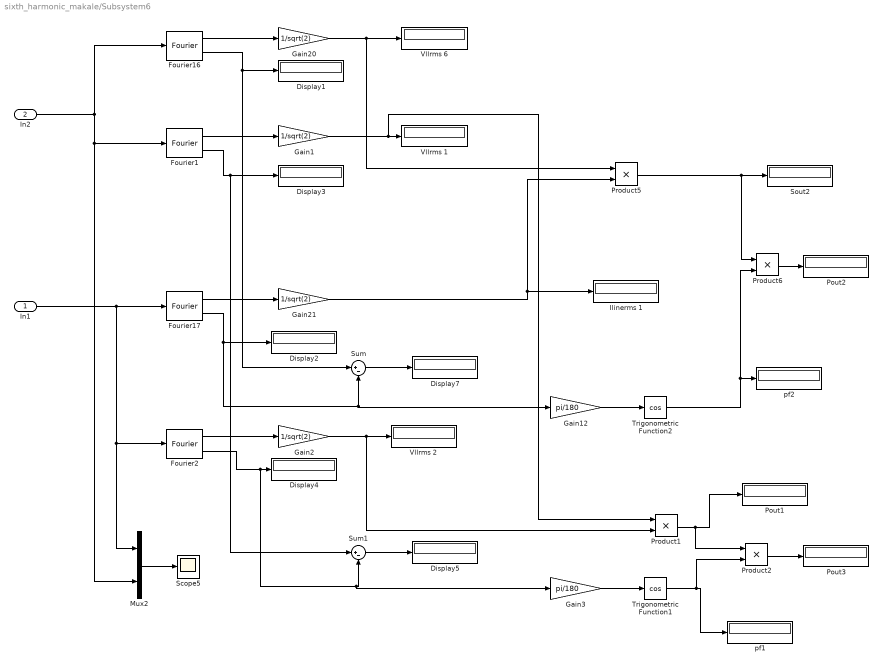
== system sixth_harmonic_makale/Subsystem6 ==
  In1 : Inport
  In2 : Inport  Port=2
  Display{1..5,7} (6 alike) : Display
  Fourier1 : powerlib_meascontrol/Measurements/Fourier  Freq=fout_fund  n=3  InInit=[0, 0]  Ts=Ts
  Fourier16 : powerlib_meascontrol/Measurements/Fourier  Freq=fout_fund  n=1  InInit=[0, 0]  Ts=Ts
  Fourier17 : powerlib_meascontrol/Measurements/Fourier  Freq=fout_fund  n=1  InInit=[0, 0]  Ts=Ts
  Fourier2 : powerlib_meascontrol/Measurements/Fourier  Freq=fout_fund  n=3  InInit=[0, 0]  Ts=Ts
  Gain{1..2,20..21} (4 alike) : Gain  Gain=1/sqrt(2)
  Gain12 : Gain  Gain=pi/180
  Gain3 : Gain  Gain=pi/180
  Ilinerms 1 : Display
  Mux2 : Mux  Inputs=2
  Pout1 : Display
  Pout2 : Display
  Pout3 : Display
  Product{1..2,5..6} (4 alike) : Product
  Scope5 : Scope
      settings: YMin=-700  YMax=700  SaveName=ScopeData2
  Sout2 : Display
      settings: Format=short_e
  Sum : Sum  Inputs=|+-
  Sum1 : Sum  Inputs=|+-
  Trigonometric Function1 : Trigonometry  Operator=cos
  Trigonometric Function2 : Trigonometry  Operator=cos
  Vllrms 1 : Display
  Vllrms 2 : Display
  Vllrms 6 : Display
  pf1 : Display
  pf2 : Display
  wires:
  Mux2/1 -> Scope5/1
  In2/1 -> Fourier16/1, Fourier1/1, Mux2/2
  In1/1 -> Fourier17/1, Fourier2/1, Mux2/1
  Gain20/1 -> Vllrms 6/1, Product5/1
  Gain21/1 -> Ilinerms 1/1, Product5/2
  Fourier17/1 -> Gain21/1
  Trigonometric Function2/1 -> Product6/2, pf2/1
  Gain12/1 -> Trigonometric Function2/1
  Product6/1 -> Pout2/1
  Fourier16/1 -> Gain20/1
  Product5/1 -> Product6/1, Sout2/1
  Fourier16/2 -> Display1/1, Sum/1
  Fourier17/2 -> Display2/1, Sum/2, Gain12/1
  Sum/1 -> Display7/1
  Fourier1/1 -> Gain1/1
  Gain1/1 -> Product1/1, Vllrms 1/1
  Fourier1/2 -> Display3/1, Sum1/1
  Fourier2/1 -> Gain2/1
  Gain2/1 -> Product1/2, Vllrms 2/1
  Fourier2/2 -> Gain3/1, Sum1/2, Display4/1
  Sum1/1 -> Display5/1
  Gain3/1 -> Trigonometric Function1/1
  Trigonometric Function1/1 -> Product2/2, pf1/1
  Product1/1 -> Product2/1, Pout1/1
  Product2/1 -> Pout3/1

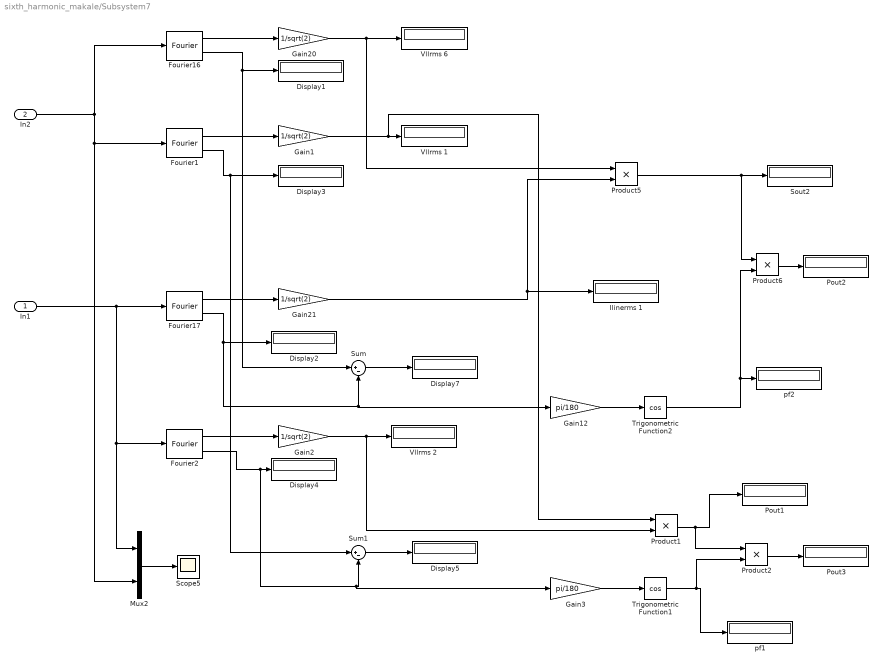
== system sixth_harmonic_makale/Subsystem7 ==
  In1 : Inport
  In2 : Inport  Port=2
  Display{1..5,7} (6 alike) : Display
  Fourier1 : powerlib_meascontrol/Measurements/Fourier  Freq=fout_fund  n=3  InInit=[0, 0]  Ts=Ts
  Fourier16 : powerlib_meascontrol/Measurements/Fourier  Freq=fout_fund  n=1  InInit=[0, 0]  Ts=Ts
  Fourier17 : powerlib_meascontrol/Measurements/Fourier  Freq=fout_fund  n=1  InInit=[0, 0]  Ts=Ts
  Fourier2 : powerlib_meascontrol/Measurements/Fourier  Freq=fout_fund  n=3  InInit=[0, 0]  Ts=Ts
  Gain{1..2,20..21} (4 alike) : Gain  Gain=1/sqrt(2)
  Gain12 : Gain  Gain=pi/180
  Gain3 : Gain  Gain=pi/180
  Ilinerms 1 : Display
  Mux2 : Mux  Inputs=2
  Pout1 : Display
  Pout2 : Display
  Pout3 : Display
  Product{1..2,5..6} (4 alike) : Product
  Scope5 : Scope
      settings: YMin=-700  YMax=700  SaveName=ScopeData2
  Sout2 : Display
      settings: Format=short_e
  Sum : Sum  Inputs=|+-
  Sum1 : Sum  Inputs=|+-
  Trigonometric Function1 : Trigonometry  Operator=cos
  Trigonometric Function2 : Trigonometry  Operator=cos
  Vllrms 1 : Display
  Vllrms 2 : Display
  Vllrms 6 : Display
  pf1 : Display
  pf2 : Display
  wires:
  Mux2/1 -> Scope5/1
  In2/1 -> Fourier16/1, Fourier1/1, Mux2/2
  In1/1 -> Fourier17/1, Fourier2/1, Mux2/1
  Gain20/1 -> Vllrms 6/1, Product5/1
  Gain21/1 -> Ilinerms 1/1, Product5/2
  Fourier17/1 -> Gain21/1
  Trigonometric Function2/1 -> Product6/2, pf2/1
  Gain12/1 -> Trigonometric Function2/1
  Product6/1 -> Pout2/1
  Fourier16/1 -> Gain20/1
  Product5/1 -> Product6/1, Sout2/1
  Fourier16/2 -> Display1/1, Sum/1
  Fourier17/2 -> Display2/1, Sum/2, Gain12/1
  Sum/1 -> Display7/1
  Fourier1/1 -> Gain1/1
  Gain1/1 -> Product1/1, Vllrms 1/1
  Fourier1/2 -> Display3/1, Sum1/1
  Fourier2/1 -> Gain2/1
  Gain2/1 -> Product1/2, Vllrms 2/1
  Fourier2/2 -> Gain3/1, Sum1/2, Display4/1
  Sum1/1 -> Display5/1
  Gain3/1 -> Trigonometric Function1/1
  Trigonometric Function1/1 -> Product2/2, pf1/1
  Product1/1 -> Product2/1, Pout1/1
  Product2/1 -> Pout3/1

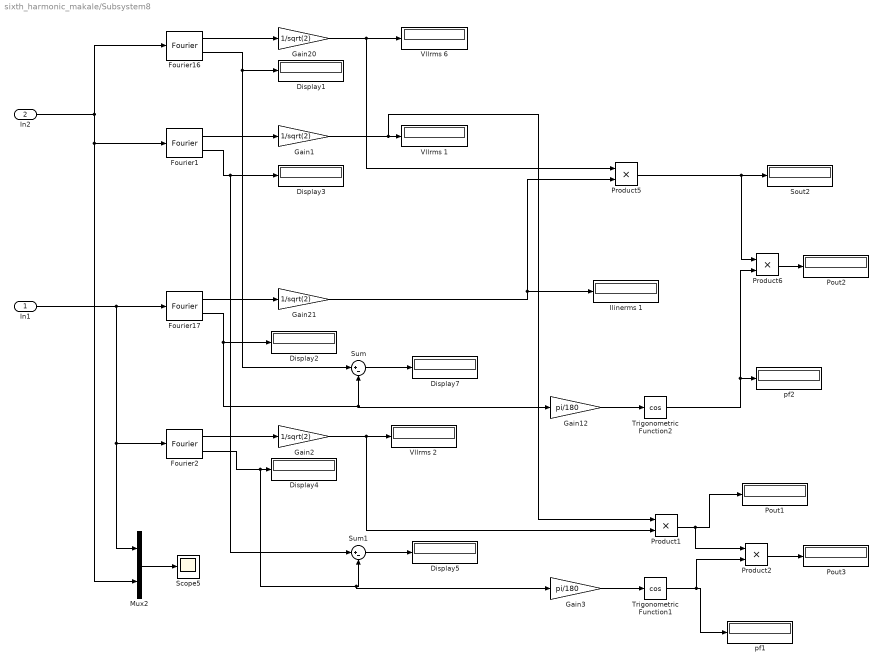
== system sixth_harmonic_makale/Subsystem8 ==
  In1 : Inport
  In2 : Inport  Port=2
  Display{1..5,7} (6 alike) : Display
  Fourier1 : powerlib_meascontrol/Measurements/Fourier  Freq=fout_fund  n=3  InInit=[0, 0]  Ts=Ts
  Fourier16 : powerlib_meascontrol/Measurements/Fourier  Freq=fout_fund  n=1  InInit=[0, 0]  Ts=Ts
  Fourier17 : powerlib_meascontrol/Measurements/Fourier  Freq=fout_fund  n=1  InInit=[0, 0]  Ts=Ts
  Fourier2 : powerlib_meascontrol/Measurements/Fourier  Freq=fout_fund  n=3  InInit=[0, 0]  Ts=Ts
  Gain{1..2,20..21} (4 alike) : Gain  Gain=1/sqrt(2)
  Gain12 : Gain  Gain=pi/180
  Gain3 : Gain  Gain=pi/180
  Ilinerms 1 : Display
  Mux2 : Mux  Inputs=2
  Pout1 : Display
  Pout2 : Display
  Pout3 : Display
  Product{1..2,5..6} (4 alike) : Product
  Scope5 : Scope
      settings: YMin=-700  YMax=700  SaveName=ScopeData2
  Sout2 : Display
      settings: Format=short_e
  Sum : Sum  Inputs=|+-
  Sum1 : Sum  Inputs=|+-
  Trigonometric Function1 : Trigonometry  Operator=cos
  Trigonometric Function2 : Trigonometry  Operator=cos
  Vllrms 1 : Display
  Vllrms 2 : Display
  Vllrms 6 : Display
  pf1 : Display
  pf2 : Display
  wires:
  Mux2/1 -> Scope5/1
  In2/1 -> Fourier16/1, Fourier1/1, Mux2/2
  In1/1 -> Fourier17/1, Fourier2/1, Mux2/1
  Gain20/1 -> Vllrms 6/1, Product5/1
  Gain21/1 -> Ilinerms 1/1, Product5/2
  Fourier17/1 -> Gain21/1
  Trigonometric Function2/1 -> Product6/2, pf2/1
  Gain12/1 -> Trigonometric Function2/1
  Product6/1 -> Pout2/1
  Fourier16/1 -> Gain20/1
  Product5/1 -> Product6/1, Sout2/1
  Fourier16/2 -> Display1/1, Sum/1
  Fourier17/2 -> Display2/1, Sum/2, Gain12/1
  Sum/1 -> Display7/1
  Fourier1/1 -> Gain1/1
  Gain1/1 -> Product1/1, Vllrms 1/1
  Fourier1/2 -> Display3/1, Sum1/1
  Fourier2/1 -> Gain2/1
  Gain2/1 -> Product1/2, Vllrms 2/1
  Fourier2/2 -> Gain3/1, Sum1/2, Display4/1
  Sum1/1 -> Display5/1
  Gain3/1 -> Trigonometric Function1/1
  Trigonometric Function1/1 -> Product2/2, pf1/1
  Product1/1 -> Product2/1, Pout1/1
  Product2/1 -> Pout3/1

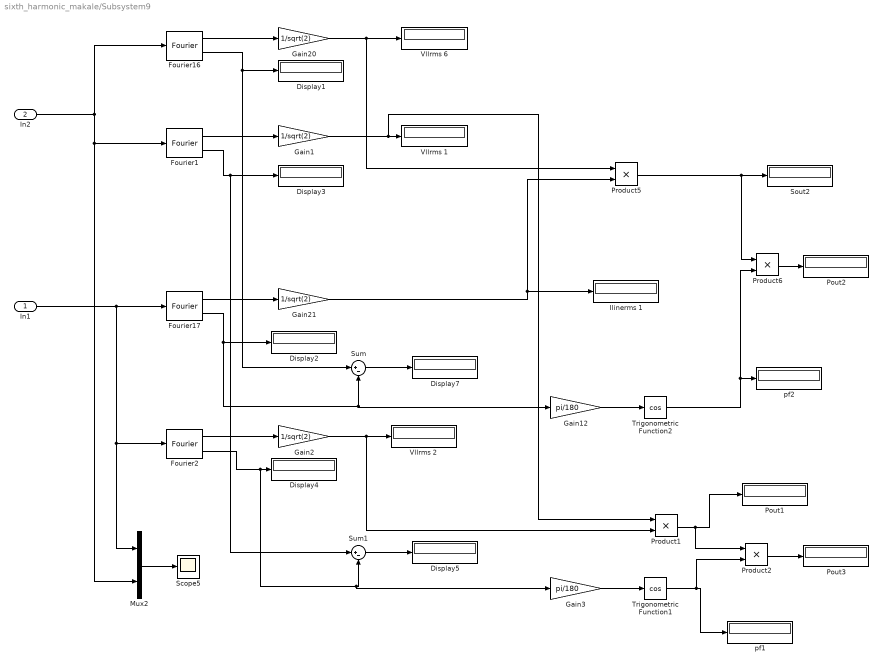
== system sixth_harmonic_makale/Subsystem9 ==
  In1 : Inport
  In2 : Inport  Port=2
  Display{1..5,7} (6 alike) : Display
  Fourier1 : powerlib_meascontrol/Measurements/Fourier  Freq=fout_fund  n=3  InInit=[0, 0]  Ts=Ts
  Fourier16 : powerlib_meascontrol/Measurements/Fourier  Freq=fout_fund  n=1  InInit=[0, 0]  Ts=Ts
  Fourier17 : powerlib_meascontrol/Measurements/Fourier  Freq=fout_fund  n=1  InInit=[0, 0]  Ts=Ts
  Fourier2 : powerlib_meascontrol/Measurements/Fourier  Freq=fout_fund  n=3  InInit=[0, 0]  Ts=Ts
  Gain{1..2,20..21} (4 alike) : Gain  Gain=1/sqrt(2)
  Gain12 : Gain  Gain=pi/180
  Gain3 : Gain  Gain=pi/180
  Ilinerms 1 : Display
  Mux2 : Mux  Inputs=2
  Pout1 : Display
  Pout2 : Display
  Pout3 : Display
  Product{1..2,5..6} (4 alike) : Product
  Scope5 : Scope
      settings: YMin=-700  YMax=700  SaveName=ScopeData2
  Sout2 : Display
      settings: Format=short_e
  Sum : Sum  Inputs=|+-
  Sum1 : Sum  Inputs=|+-
  Trigonometric Function1 : Trigonometry  Operator=cos
  Trigonometric Function2 : Trigonometry  Operator=cos
  Vllrms 1 : Display
  Vllrms 2 : Display
  Vllrms 6 : Display
  pf1 : Display
  pf2 : Display
  wires:
  Mux2/1 -> Scope5/1
  In2/1 -> Fourier16/1, Fourier1/1, Mux2/2
  In1/1 -> Fourier17/1, Fourier2/1, Mux2/1
  Gain20/1 -> Vllrms 6/1, Product5/1
  Gain21/1 -> Ilinerms 1/1, Product5/2
  Fourier17/1 -> Gain21/1
  Trigonometric Function2/1 -> Product6/2, pf2/1
  Gain12/1 -> Trigonometric Function2/1
  Product6/1 -> Pout2/1
  Fourier16/1 -> Gain20/1
  Product5/1 -> Product6/1, Sout2/1
  Fourier16/2 -> Display1/1, Sum/1
  Fourier17/2 -> Display2/1, Sum/2, Gain12/1
  Sum/1 -> Display7/1
  Fourier1/1 -> Gain1/1
  Gain1/1 -> Product1/1, Vllrms 1/1
  Fourier1/2 -> Display3/1, Sum1/1
  Fourier2/1 -> Gain2/1
  Gain2/1 -> Product1/2, Vllrms 2/1
  Fourier2/2 -> Gain3/1, Sum1/2, Display4/1
  Sum1/1 -> Display5/1
  Gain3/1 -> Trigonometric Function1/1
  Trigonometric Function1/1 -> Product2/2, pf1/1
  Product1/1 -> Product2/1, Pout1/1
  Product2/1 -> Pout3/1
